simulink model "controle_estabilidade_2"  (R2021b)
settings: Solver=ode45  StartTime=0.0  StopTime=30.0  MaxStep=0.4  RelTol=1e-3
values from neighbouring files (symbols this model uses):
  B = 8.85e-06    [parametros2.mat]
  b = 5.16e-06    [parametros.mat]    (also in parametros2.mat)
  J = [0.00216966666667  0  0; 0  0.00216966666667  0; 0  0  0.00216966666667]    [parametros.mat]    (also in parametros2.mat)
  J_m = 3e-06    [parametros2.mat]
  Jr = 3e-06    [parametros.mat]    (also in parametros2.mat)
  kd = 0    [parametros2.mat]
  Ke = 0.000922    [parametros2.mat]
  ki = 0    [parametros2.mat]
  Kiw = 0.04667    [parametros.mat]    (also in parametros2.mat = 0.0467)
  Km = 0.0264    [parametros.mat]    (also in parametros2.mat)
  kp = 1    [parametros2.mat]
  Kpw = 0.17718    [parametros.mat]    (also in parametros2.mat = 0.1772)
  Kt = 0.0088    [parametros2.mat]
  L_a = 0.48    [parametros2.mat]
  R_a = 7    [parametros2.mat]
libraries: slpidlib x4, sharedutil x1, aerolibutil x1
settings Model: Creator=JRRL  LastModifiedBy=JRRL

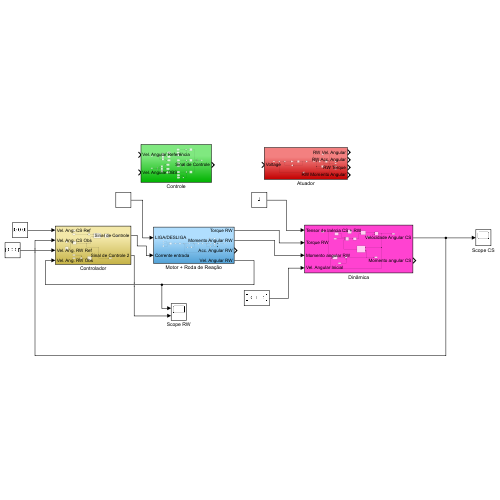
[thumbnail: Simulink's stored preview of the top-level diagram]
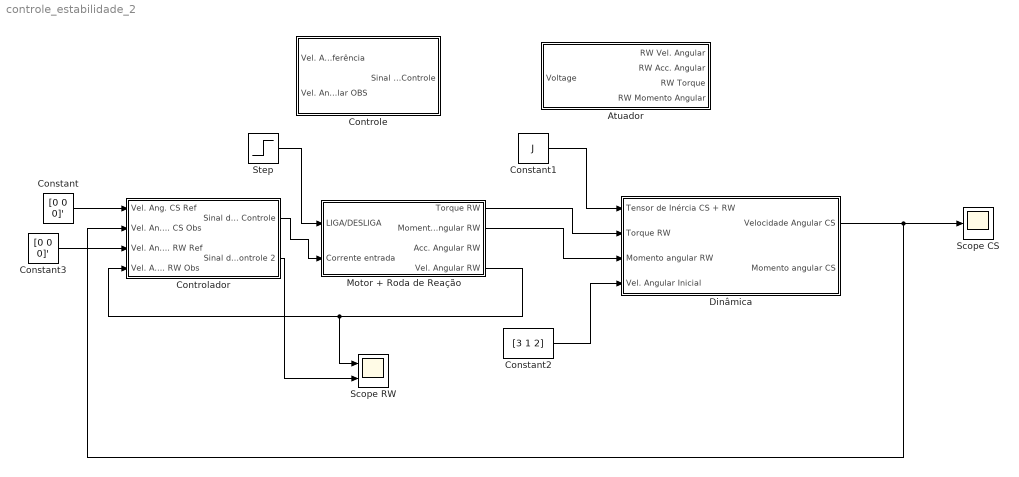
== system controle_estabilidade_2 ==
  Atuador : Subsystem
  Constant : Constant  Value=[0 0 0]'
  Constant1 : Constant  Value=J
  Constant2 : Constant  Value=[3 1 2]
  Constant3 : Constant  Value=[0 0 0]'
  Controlador : Subsystem
  Controle : Subsystem
  Dinâmica : Subsystem
  Motor + Roda de Reação : Subsystem
  Scope CS : Scope
  Scope RW : Scope  NumInputPorts=2
  Step : Step  Time=50  Before=1  After=0  SampleTime=0
  wires:
  Constant1/1 -> Dinâmica/1(Tensor de Inércia CS + RW)
  Dinâmica/1(Velocidade Angular CS) -> Controlador/2(Vel. Ang. CS Obs), Scope CS/1
  Constant/1 -> Controlador/1(Vel. Ang. CS Ref)
  Motor + Roda de Reação/1(Torque RW) -> Dinâmica/2(Torque RW)
  Motor + Roda de Reação/2(Momento Angular RW) -> Dinâmica/3(Momento angular RW)
  Constant2/1 -> Dinâmica/4(Vel. Angular Inicial)
  Motor + Roda de Reação/4(Vel. Angular RW) -> Scope RW/1, Controlador/4(Vel. Ang. RW Obs)
  Step/1 -> Motor + Roda de Reação/1(LIGA/DESLIGA)
  Controlador/1(Sinal de Controle) -> Motor + Roda de Reação/2(Corrente entrada)
  Constant3/1 -> Controlador/3(Vel. Ang. RW Ref)
  Controlador/2(Sinal de Controle 2) -> Scope RW/2

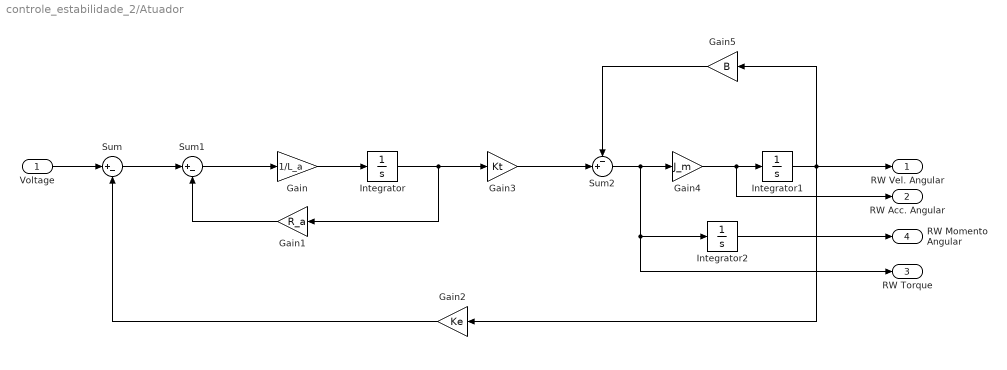
== system controle_estabilidade_2/Atuador ==
  Voltage : Inport
  Gain : Gain  Gain=1/L_a
  Gain1 : Gain  Gain=R_a
  Gain2 : Gain  Gain=Ke
  Gain3 : Gain  Gain=Kt
  Gain4 : Gain  Gain=J_m
  Gain5 : Gain  Gain=B
  Integrator : Integrator
  Integrator1 : Integrator
  Integrator2 : Integrator
  Sum : Sum  Inputs=|+-
  Sum1 : Sum  Inputs=|+-
  Sum2 : Sum  Inputs=-+|
  RW Vel. Angular : Outport
  RW Acc. Angular : Outport  Port=2
  RW Torque : Outport  Port=3
  RW Momento Angular : Outport  Port=4
  wires:
  Integrator1/1 -> RW Vel. Angular/1, Gain5/1, Gain2/1
  Gain4/1 -> RW Acc. Angular/1, Integrator1/1
  Sum2/1 -> RW Torque/1, Integrator2/1, Gain4/1
  Gain3/1 -> Sum2/2
  Integrator/1 -> Gain1/1, Gain3/1
  Voltage/1 -> Sum/1
  Sum/1 -> Sum1/1
  Gain/1 -> Integrator/1
  Sum1/1 -> Gain/1
  Gain5/1 -> Sum2/1
  Gain2/1 -> Sum/2
  Gain1/1 -> Sum1/2
  Integrator2/1 -> RW Momento Angular/1

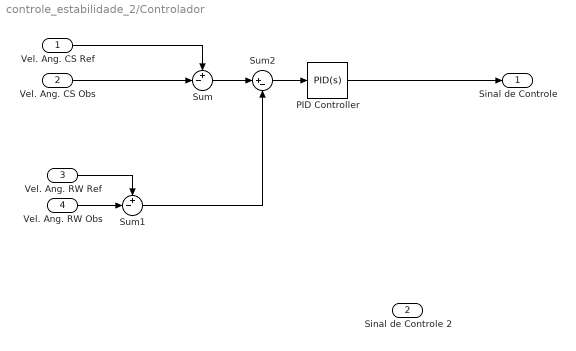
== system controle_estabilidade_2/Controlador ==
  Vel. Ang. CS Ref : Inport
  Vel. Ang. CS Obs : Inport  Port=2
  Vel. Ang. RW Ref : Inport  Port=3
  Vel. Ang. RW Obs : Inport  Port=4
  PID Controller : slpidlib/PID Controller  Controller=PID  Form=Parallel  TimeDomain=Continuous-time  UseExternalTs=off  SampleTime=-1  IntegratorMethod=Forward Euler  FilterMethod=Forward Euler  ControllerParametersSource=internal  P=1  I=1  D=0  UseFilter=on  N=100  TunerSelectOption=Transfer Function Based (PID Tuner App)  InitialConditionSource=internal  InitialConditionForIntegrator=0  InitialConditionForFilter=0  DifferentiatorICPrevScaledInput=0  ExternalReset=none  TrackingMode=off  Kt=1  LimitOutput=off  SatLimitsSource=internal  UpperSaturationLimit=inf  LowerSaturationLimit=-inf  LinearizeAsGain=on  AntiWindupMode=none  Kb=1  POutMin=[]  POutMax=[]  IOutMin=[]  IOutMax=[]  DOutMin=[]  DOutMax=[]  NOutMin=[]  NOutMax=[]  SumOutMin=[]  SumOutMax=[]  SaturationOutMin=[]  SaturationOutMax=[]  PParamMin=[]  PParamMax=[]  IParamMin=[]  IParamMax=[]  DParamMin=[]  DParamMax=[]  NParamMin=[]  NParamMax=[]  KbParamMin=[]  KbParamMax=[]  KtParamMin=[]  KtParamMax=[]  KbOutMin=[]  KbOutMax=[]  KtOutMin=[]  KtOutMax=[]  IntegratorOutMin=[]  IntegratorOutMax=[]  FilterOutMin=[]  FilterOutMax=[]  SumI1OutMin=[]  SumI1OutMax=[]  SumI2OutMin=[]  SumI2OutMax=[]  SumI3OutMin=[]  SumI3OutMax=[]  SumI4OutMin=[]  SumI4OutMax=[]  SumDOutMin=[]  SumDOutMax=[]  DifferentiatorOutMin=[]  DifferentiatorOutMax=[]  FilterDiffOutCoefMin=[]  FilterDiffOutCoefMax=[]  ReciprocalOutMin=[]  ReciprocalOutMax=[]  SumDenOutMin=[]  SumDenOutMax=[]  SumNumOutMin=[]  SumNumOutMax=[]  DivideOutMin=[]  DivideOutMax=[]  UdiffTsProdOutMin=[]  UdiffTsProdOutMax=[]  NTsProdOutMin=[]  NTsProdOutMax=[]  UintegralTsProdOutMin=[]  UintegralTsProdOutMax=[]  UngainTsProdOutMin=[]  UngainTsProdOutMax=[]  IntegratorContinuousStateAttributes=''  IntegratorStateMustResolveToSignalObject=off  IntegratorRTWStateStorageClass=Auto  FilterContinuousStateAttributes=''  FilterStateMustResolveToSignalObject=off  FilterRTWStateStorageClass=Auto  ParallelPVariant=InternalParameters  IdealPVariant=Disabled  IVariant=InternalParameters  DVariant=InternalParameters  IntegratorVariant=Continuous  SatVariant=Disabled  AWVariant=Passthrough  PCopyVariant=Disabled  TRVariant=Disabled  FdbkBlocksVariant=Forward  IdealPFdbkVariant=Disabled  SatFdbkVariant=Disabled  DerivativeFilterVariant=ContFilter  NVariant=InternalParameters  NCopyVariant=Disabled  FilterICVariant=InternalICsFilter  IntegratorICVariant=InternalICs  ExternalResetVariant=Disabled  TRSumVariant=Passthrough  SumFdbkVariant=Disabled  SumVariant=Sum_PID  TsampFilterVariant=InternalTs  TsampNgainVariant=Passthrough  TsampIntegralVariant=Passthrough  ExternalSaturationOutDataTypeStr=Inherit: Same as second input
  Sum : Sum  Inputs=+-|
  Sum1 : Sum  Inputs=+-|
  Sum2 : Sum  Inputs=|+-
  Sinal de Controle : Outport
  Sinal de Controle 2 : Outport  Port=2
  wires:
  Vel. Ang. CS Ref/1 -> Sum/1
  Vel. Ang. CS Obs/1 -> Sum/2
  Vel. Ang. RW Ref/1 -> Sum1/1
  Vel. Ang. RW Obs/1 -> Sum1/2
  Sum1/1 -> Sum2/2
  PID Controller/1 -> Sinal de Controle/1
  Sum/1 -> Sum2/1
  Sum2/1 -> PID Controller/1

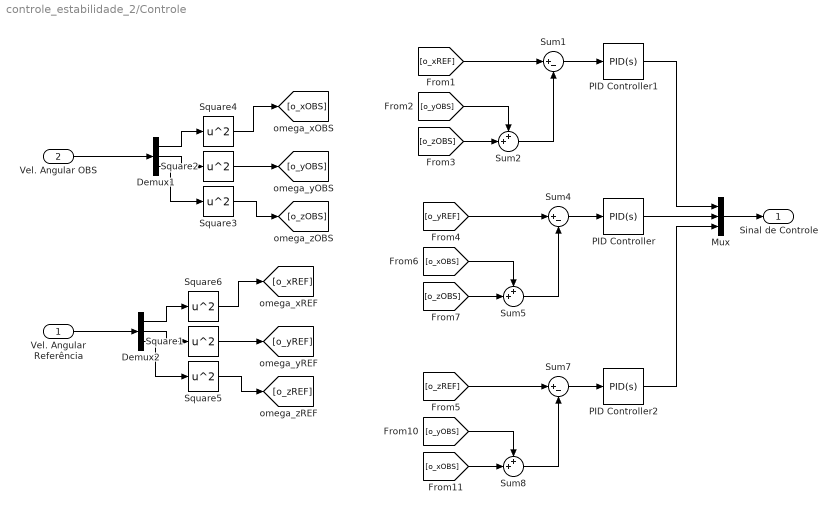
== system controle_estabilidade_2/Controle ==
  Vel. Angular Referência : Inport
  Vel. Angular OBS : Inport  Port=2
  Demux1 : Demux  Outputs=3
  Demux2 : Demux  Outputs=3
  Mux : Mux  Inputs=3
  PID Controller : slpidlib/PID Controller  Controller=PID  Form=Parallel  TimeDomain=Continuous-time  UseExternalTs=off  SampleTime=-1  IntegratorMethod=Forward Euler  FilterMethod=Forward Euler  ControllerParametersSource=internal  P=kp  I=ki  D=kd  UseFilter=on  N=100  TunerSelectOption=Transfer Function Based (PID Tuner App)  InitialConditionSource=internal  InitialConditionForIntegrator=0  InitialConditionForFilter=0  DifferentiatorICPrevScaledInput=0  ExternalReset=none  TrackingMode=off  Kt=1  LimitOutput=off  SatLimitsSource=internal  UpperSaturationLimit=inf  LowerSaturationLimit=-inf  LinearizeAsGain=on  AntiWindupMode=none  Kb=1  POutMin=[]  POutMax=[]  IOutMin=[]  IOutMax=[]  DOutMin=[]  DOutMax=[]  NOutMin=[]  NOutMax=[]  SumOutMin=[]  SumOutMax=[]  SaturationOutMin=[]  SaturationOutMax=[]  PParamMin=[]  PParamMax=[]  IParamMin=[]  IParamMax=[]  DParamMin=[]  DParamMax=[]  NParamMin=[]  NParamMax=[]  KbParamMin=[]  KbParamMax=[]  KtParamMin=[]  KtParamMax=[]  KbOutMin=[]  KbOutMax=[]  KtOutMin=[]  KtOutMax=[]  IntegratorOutMin=[]  IntegratorOutMax=[]  FilterOutMin=[]  FilterOutMax=[]  SumI1OutMin=[]  SumI1OutMax=[]  SumI2OutMin=[]  SumI2OutMax=[]  SumI3OutMin=[]  SumI3OutMax=[]  SumI4OutMin=[]  SumI4OutMax=[]  SumDOutMin=[]  SumDOutMax=[]  DifferentiatorOutMin=[]  DifferentiatorOutMax=[]  FilterDiffOutCoefMin=[]  FilterDiffOutCoefMax=[]  ReciprocalOutMin=[]  ReciprocalOutMax=[]  SumDenOutMin=[]  SumDenOutMax=[]  SumNumOutMin=[]  SumNumOutMax=[]  DivideOutMin=[]  DivideOutMax=[]  UdiffTsProdOutMin=[]  UdiffTsProdOutMax=[]  NTsProdOutMin=[]  NTsProdOutMax=[]  UintegralTsProdOutMin=[]  UintegralTsProdOutMax=[]  UngainTsProdOutMin=[]  UngainTsProdOutMax=[]  IntegratorContinuousStateAttributes=''  IntegratorStateMustResolveToSignalObject=off  IntegratorRTWStateStorageClass=Auto  FilterContinuousStateAttributes=''  FilterStateMustResolveToSignalObject=off  FilterRTWStateStorageClass=Auto  ParallelPVariant=InternalParameters  IdealPVariant=Disabled  IVariant=InternalParameters  DVariant=InternalParameters  IntegratorVariant=Continuous  SatVariant=Disabled  AWVariant=Passthrough  PCopyVariant=Disabled  TRVariant=Disabled  FdbkBlocksVariant=Forward  IdealPFdbkVariant=Disabled  SatFdbkVariant=Disabled  DerivativeFilterVariant=ContFilter  NVariant=InternalParameters  NCopyVariant=Disabled  FilterICVariant=InternalICsFilter  IntegratorICVariant=InternalICs  ExternalResetVariant=Disabled  TRSumVariant=Passthrough  SumFdbkVariant=Disabled  SumVariant=Sum_PID  TsampFilterVariant=InternalTs  TsampNgainVariant=Passthrough  TsampIntegralVariant=Passthrough  ExternalSaturationOutDataTypeStr=Inherit: Same as second input
  PID Controller1 : slpidlib/PID Controller  Controller=PID  Form=Parallel  TimeDomain=Continuous-time  UseExternalTs=off  SampleTime=-1  IntegratorMethod=Forward Euler  FilterMethod=Forward Euler  ControllerParametersSource=internal  P=kp  I=ki  D=kd  UseFilter=on  N=100  TunerSelectOption=Transfer Function Based (PID Tuner App)  InitialConditionSource=internal  InitialConditionForIntegrator=0  InitialConditionForFilter=0  DifferentiatorICPrevScaledInput=0  ExternalReset=none  TrackingMode=off  Kt=1  LimitOutput=off  SatLimitsSource=internal  UpperSaturationLimit=inf  LowerSaturationLimit=-inf  LinearizeAsGain=on  AntiWindupMode=none  Kb=1  POutMin=[]  POutMax=[]  IOutMin=[]  IOutMax=[]  DOutMin=[]  DOutMax=[]  NOutMin=[]  NOutMax=[]  SumOutMin=[]  SumOutMax=[]  SaturationOutMin=[]  SaturationOutMax=[]  PParamMin=[]  PParamMax=[]  IParamMin=[]  IParamMax=[]  DParamMin=[]  DParamMax=[]  NParamMin=[]  NParamMax=[]  KbParamMin=[]  KbParamMax=[]  KtParamMin=[]  KtParamMax=[]  KbOutMin=[]  KbOutMax=[]  KtOutMin=[]  KtOutMax=[]  IntegratorOutMin=[]  IntegratorOutMax=[]  FilterOutMin=[]  FilterOutMax=[]  SumI1OutMin=[]  SumI1OutMax=[]  SumI2OutMin=[]  SumI2OutMax=[]  SumI3OutMin=[]  SumI3OutMax=[]  SumI4OutMin=[]  SumI4OutMax=[]  SumDOutMin=[]  SumDOutMax=[]  DifferentiatorOutMin=[]  DifferentiatorOutMax=[]  FilterDiffOutCoefMin=[]  FilterDiffOutCoefMax=[]  ReciprocalOutMin=[]  ReciprocalOutMax=[]  SumDenOutMin=[]  SumDenOutMax=[]  SumNumOutMin=[]  SumNumOutMax=[]  DivideOutMin=[]  DivideOutMax=[]  UdiffTsProdOutMin=[]  UdiffTsProdOutMax=[]  NTsProdOutMin=[]  NTsProdOutMax=[]  UintegralTsProdOutMin=[]  UintegralTsProdOutMax=[]  UngainTsProdOutMin=[]  UngainTsProdOutMax=[]  IntegratorContinuousStateAttributes=''  IntegratorStateMustResolveToSignalObject=off  IntegratorRTWStateStorageClass=Auto  FilterContinuousStateAttributes=''  FilterStateMustResolveToSignalObject=off  FilterRTWStateStorageClass=Auto  ParallelPVariant=InternalParameters  IdealPVariant=Disabled  IVariant=InternalParameters  DVariant=InternalParameters  IntegratorVariant=Continuous  SatVariant=Disabled  AWVariant=Passthrough  PCopyVariant=Disabled  TRVariant=Disabled  FdbkBlocksVariant=Forward  IdealPFdbkVariant=Disabled  SatFdbkVariant=Disabled  DerivativeFilterVariant=ContFilter  NVariant=InternalParameters  NCopyVariant=Disabled  FilterICVariant=InternalICsFilter  IntegratorICVariant=InternalICs  ExternalResetVariant=Disabled  TRSumVariant=Passthrough  SumFdbkVariant=Disabled  SumVariant=Sum_PID  TsampFilterVariant=InternalTs  TsampNgainVariant=Passthrough  TsampIntegralVariant=Passthrough  ExternalSaturationOutDataTypeStr=Inherit: Same as second input
  PID Controller2 : slpidlib/PID Controller  Controller=PID  Form=Parallel  TimeDomain=Continuous-time  UseExternalTs=off  SampleTime=-1  IntegratorMethod=Forward Euler  FilterMethod=Forward Euler  ControllerParametersSource=internal  P=kp  I=ki  D=kd  UseFilter=on  N=100  TunerSelectOption=Transfer Function Based (PID Tuner App)  InitialConditionSource=internal  InitialConditionForIntegrator=0  InitialConditionForFilter=0  DifferentiatorICPrevScaledInput=0  ExternalReset=none  TrackingMode=off  Kt=1  LimitOutput=off  SatLimitsSource=internal  UpperSaturationLimit=inf  LowerSaturationLimit=-inf  LinearizeAsGain=on  AntiWindupMode=none  Kb=1  POutMin=[]  POutMax=[]  IOutMin=[]  IOutMax=[]  DOutMin=[]  DOutMax=[]  NOutMin=[]  NOutMax=[]  SumOutMin=[]  SumOutMax=[]  SaturationOutMin=[]  SaturationOutMax=[]  PParamMin=[]  PParamMax=[]  IParamMin=[]  IParamMax=[]  DParamMin=[]  DParamMax=[]  NParamMin=[]  NParamMax=[]  KbParamMin=[]  KbParamMax=[]  KtParamMin=[]  KtParamMax=[]  KbOutMin=[]  KbOutMax=[]  KtOutMin=[]  KtOutMax=[]  IntegratorOutMin=[]  IntegratorOutMax=[]  FilterOutMin=[]  FilterOutMax=[]  SumI1OutMin=[]  SumI1OutMax=[]  SumI2OutMin=[]  SumI2OutMax=[]  SumI3OutMin=[]  SumI3OutMax=[]  SumI4OutMin=[]  SumI4OutMax=[]  SumDOutMin=[]  SumDOutMax=[]  DifferentiatorOutMin=[]  DifferentiatorOutMax=[]  FilterDiffOutCoefMin=[]  FilterDiffOutCoefMax=[]  ReciprocalOutMin=[]  ReciprocalOutMax=[]  SumDenOutMin=[]  SumDenOutMax=[]  SumNumOutMin=[]  SumNumOutMax=[]  DivideOutMin=[]  DivideOutMax=[]  UdiffTsProdOutMin=[]  UdiffTsProdOutMax=[]  NTsProdOutMin=[]  NTsProdOutMax=[]  UintegralTsProdOutMin=[]  UintegralTsProdOutMax=[]  UngainTsProdOutMin=[]  UngainTsProdOutMax=[]  IntegratorContinuousStateAttributes=''  IntegratorStateMustResolveToSignalObject=off  IntegratorRTWStateStorageClass=Auto  FilterContinuousStateAttributes=''  FilterStateMustResolveToSignalObject=off  FilterRTWStateStorageClass=Auto  ParallelPVariant=InternalParameters  IdealPVariant=Disabled  IVariant=InternalParameters  DVariant=InternalParameters  IntegratorVariant=Continuous  SatVariant=Disabled  AWVariant=Passthrough  PCopyVariant=Disabled  TRVariant=Disabled  FdbkBlocksVariant=Forward  IdealPFdbkVariant=Disabled  SatFdbkVariant=Disabled  DerivativeFilterVariant=ContFilter  NVariant=InternalParameters  NCopyVariant=Disabled  FilterICVariant=InternalICsFilter  IntegratorICVariant=InternalICs  ExternalResetVariant=Disabled  TRSumVariant=Passthrough  SumFdbkVariant=Disabled  SumVariant=Sum_PID  TsampFilterVariant=InternalTs  TsampNgainVariant=Passthrough  TsampIntegralVariant=Passthrough  ExternalSaturationOutDataTypeStr=Inherit: Same as second input
  Square{1..6} (6 alike) : Math  Operator=square  SaturateOnIntegerOverflow=on
  Sum1 : Sum  Inputs=|+-
  Sum2 : Sum  Inputs=++|
  Sum4 : Sum  Inputs=|+-
  Sum5 : Sum  Inputs=++|
  Sum7 : Sum  Inputs=|+-
  Sum8 : Sum  Inputs=++|
  Sinal de Controle : Outport
  wires:
  Vel. Angular OBS/1 -> Demux1/1
  Demux1/2 -> Square2/1
  Demux1/3 -> Square3/1
  Demux1/1 -> Square4/1
  Square4/1 -> [o_xOBS]
  Square2/1 -> [o_yOBS]
  Square3/1 -> [o_zOBS]
  Demux2/2 -> Square1/1
  Vel. Angular Referência/1 -> Demux2/1
  Demux2/1 -> Square6/1
  Square6/1 -> [o_xREF]
  Square1/1 -> [o_yREF]
  Square5/1 -> [o_zREF]
  Demux2/3 -> Square5/1
  PID Controller1/1 -> Mux/1
  PID Controller/1 -> Mux/2
  PID Controller2/1 -> Mux/3
  Sum1/1 -> PID Controller1/1
  [o_yOBS] -> Sum2/1
  [o_zOBS] -> Sum2/2
  Sum2/1 -> Sum1/2
  Sum4/1 -> PID Controller/1
  [o_zOBS] -> Sum5/2
  [o_xOBS] -> Sum5/1
  Sum5/1 -> Sum4/2
  Sum7/1 -> PID Controller2/1
  [o_xOBS] -> Sum8/2
  [o_yOBS] -> Sum8/1
  Sum8/1 -> Sum7/2
  Mux/1 -> Sinal de Controle/1
  [o_yREF] -> Sum4/1
  [o_xREF] -> Sum1/1
  [o_zREF] -> Sum7/1

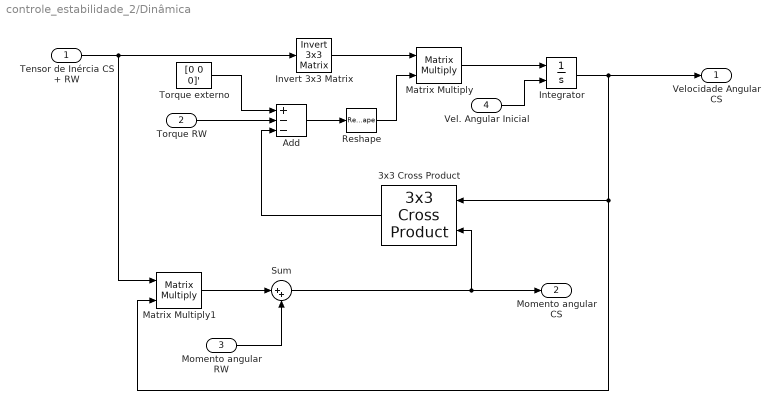
== system controle_estabilidade_2/Dinâmica ==
  Tensor de Inércia CS + RW : Inport
  Torque RW : Inport  Port=2
  Momento angular RW : Inport  Port=3
  Vel. Angular Inicial : Inport  Port=4
  3x3 Cross Product : sharedutil/3x3 Cross Product  aMode=aMode
      settings: SourceProductBaseCode=AE,PW,DR,MT,UV,VE
  Add : Sum  Inputs=+--
  Integrator : Integrator  InitialConditionSource=external
  Invert 3x3 Matrix : aerolibutil/Invert  3x3 Matrix
  Matrix Multiply : Product  Multiplication=Matrix(*)
  Matrix Multiply1 : Product  Multiplication=Matrix(*)
  Reshape : Reshape  OutputDimensionality=Column vector (2-D)
  Sum : Sum  Inputs=|++
  Torque externo : Constant  Value=[0 0 0]'
  Velocidade Angular CS : Outport
  Momento angular CS : Outport  Port=2
  wires:
  Sum/1 -> Momento angular CS/1, 3x3 Cross Product/2
  3x3 Cross Product/1 -> Add/3
  Invert 3x3 Matrix/1 -> Matrix Multiply/1
  Integrator/1 -> Velocidade Angular CS/1, Matrix Multiply1/2, 3x3 Cross Product/1
  Matrix Multiply/1 -> Integrator/1
  Momento angular RW/1 -> Sum/2
  Torque RW/1 -> Add/2
  Tensor de Inércia CS + RW/1 -> Matrix Multiply1/1, Invert 3x3 Matrix/1
  Torque externo/1 -> Add/1
  Vel. Angular Inicial/1 -> Integrator/2
  Add/1 -> Reshape/1
  Matrix Multiply1/1 -> Sum/1
  Reshape/1 -> Matrix Multiply/2

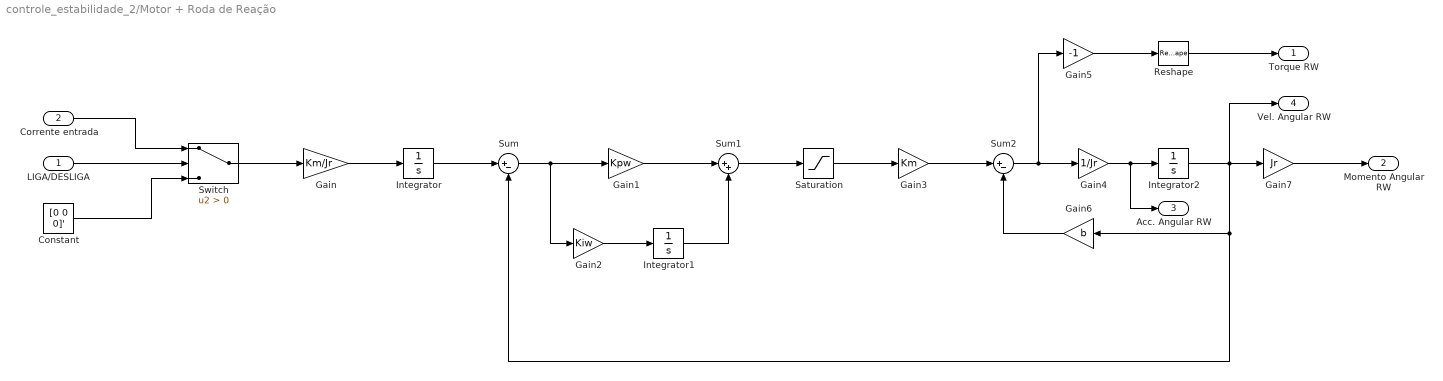
== system controle_estabilidade_2/Motor + Roda de Reação ==
  LIGA/DESLIGA : Inport
  Corrente entrada : Inport  Port=2
  Constant : Constant  Value=[0 0 0]'
  Gain : Gain  Gain=Km/Jr
  Gain1 : Gain  Gain=Kpw
  Gain2 : Gain  Gain=Kiw
  Gain3 : Gain  Gain=Km
  Gain4 : Gain  Gain=1/Jr
  Gain5 : Gain  Gain=-1
  Gain6 : Gain  Gain=b
  Gain7 : Gain  Gain=Jr
  Integrator : Integrator
  Integrator1 : Integrator
  Integrator2 : Integrator
  Reshape : Reshape  OutputDimensionality=Column vector (2-D)
  Saturation : Saturate
  Sum : Sum  Inputs=|+-
  Sum1 : Sum  Inputs=|++
  Sum2 : Sum  Inputs=|+-
  Switch : Switch  Criteria=u2 > Threshold
  Torque RW : Outport
  Momento Angular RW : Outport  Port=2
  Acc. Angular RW : Outport  Port=3
  Vel. Angular RW : Outport  Port=4
  wires:
  Saturation/1 -> Gain3/1
  Gain1/1 -> Sum1/1
  Sum/1 -> Gain2/1, Gain1/1
  Reshape/1 -> Torque RW/1
  Sum1/1 -> Saturation/1
  Gain2/1 -> Integrator1/1
  Sum2/1 -> Gain5/1, Gain4/1
  Integrator2/1 -> Vel. Angular RW/1, Sum/2, Gain6/1, Gain7/1
  Gain4/1 -> Acc. Angular RW/1, Integrator2/1
  Gain7/1 -> Momento Angular RW/1
  Gain6/1 -> Sum2/2
  Gain5/1 -> Reshape/1
  Integrator1/1 -> Sum1/2
  Gain3/1 -> Sum2/1
  Integrator/1 -> Sum/1
  Gain/1 -> Integrator/1
  LIGA/DESLIGA/1 -> Switch/2
  Corrente entrada/1 -> Switch/1
  Constant/1 -> Switch/3
  Switch/1 -> Gain/1
